simulink model "VVI"  (R2022a)
settings: Solver=FixedStepAuto  StartTime=0.0  StopTime=50  FixedStep=1e-3  RelTol=1e-3  EnableMultiTasking=on
undefined symbols (not defined in the file): D1, D10, D11, D12, D13, D2, D3, D5, D8, D9, PTA0, PTA1, PTA2, PTB9, PTC17, PTC4, PTD0, PTD1, PTD2, PTD3
libraries: frdmk64flib x10
settings Model: ExtModeTrigDuration=5  Creator=tygre  LastModifiedBy=MichaelGolendukhin
settings OptimizationCC: EnhancedBackFolding=on  PassReuseOutputArgsAs=Individual arguments  ZeroExternalMemoryAtStartup=off  ZeroInternalMemoryAtStartup=off  MaxStackSize=64  OptimizeBlockOrder=speed  DifferentSizesBufferReuse=on  OptimizationCustomize=off  EfficientTunableParamExpr=on
settings DebuggingCC: ParameterTunabilityLossMsg=error
settings HardwareCC: ProdBitPerPointer=32  ProdBitPerSizeT=32  ProdBitPerPtrDiffT=32  ProdLargestAtomicInteger=Long  ProdLargestAtomicFloat=Double  ProdWordSize=32  ProdHWDeviceType=ARM Compatible->ARM Cortex  UseEmbeddedCoderFeatures=off
settings SFSimCC: MATLABDynamicMemAlloc=off
settings RTWCC: SystemTargetFile=ert.tlc  HardwareBoard=NXP FRDM-K64F  TLCOptions="-aInlineSetEventsForThisBaseRateFcn=TLC_FALSE -aSuppressMultiTaskScheduler=TLC_FALSE  -aRateBasedStepFcn=0"  TemplateMakefile=ert_default_tmf  Toolchain=GNU Tools for ARM Embedded Processors
settings CodeAppCC: ForceParamTrailComments=on  IgnoreCustomStorageClasses=off  OperatorAnnotations=on  SimulinkDataObjDesc=on  SFDataObjDesc=on  InsertBlockDesc=on
settings ERTTargetCC: SupportNonInlinedSFcns=on  ExtModeTransport=4  ExtModeMexFile=sendToCommService

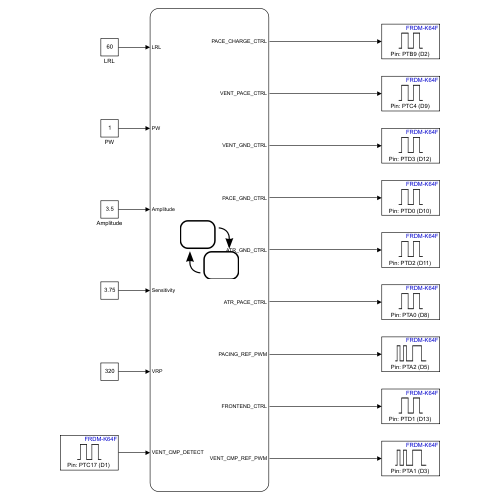
[thumbnail: Simulink's stored preview of the top-level diagram]
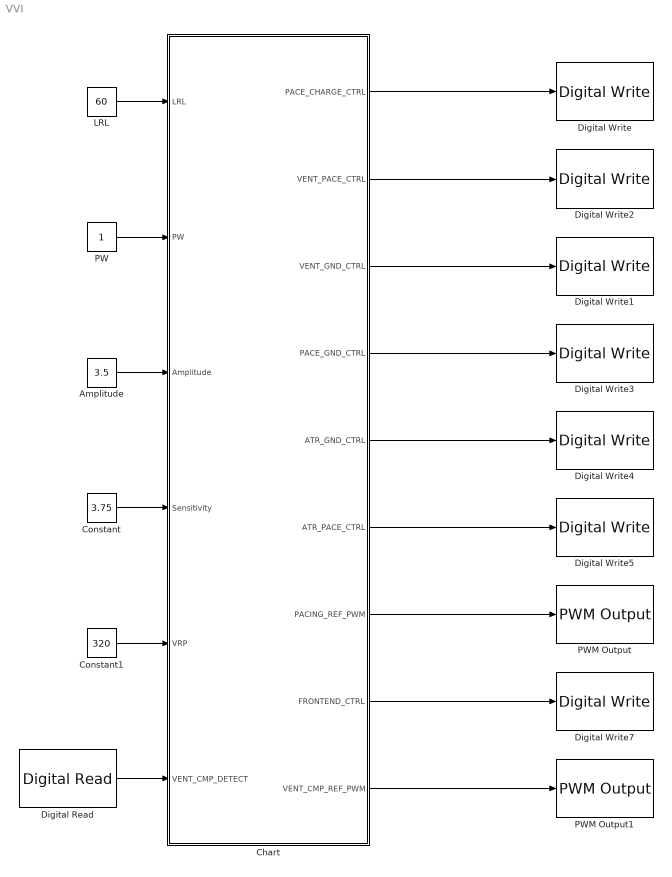
== system VVI ==
  Amplitude : Constant  Value=3.5  OutDataTypeStr=double
  Chart : Stateflow chart  TreatAsAtomicUnit=on
  Constant : Constant  Value=3.75
  Constant1 : Constant  Value=320
  Digital Read : frdmk64flib/Digital Read  Whichpin=PTC17 (D1)  SampleTime=-1
  Digital Write : frdmk64flib/Digital Write  Whichpin=PTB9 (D2)
  Digital Write1 : frdmk64flib/Digital Write  Whichpin=PTD3 (D12)
  Digital Write2 : frdmk64flib/Digital Write  Whichpin=PTC4 (D9)
  Digital Write3 : frdmk64flib/Digital Write  Whichpin=PTD0 (D10)
  Digital Write4 : frdmk64flib/Digital Write  Whichpin=PTD2 (D11)
  Digital Write5 : frdmk64flib/Digital Write  Whichpin=PTA0 (D8)
  Digital Write7 : frdmk64flib/Digital Write  Whichpin=PTD1 (D13)
  LRL : Constant  Value=60
  PW : Constant
  PWM Output : frdmk64flib/PWM Output  Whichpin=PTA2 (D5)  InitialFrequency=2000  InitialDutyCycle=0
  PWM Output1 : frdmk64flib/PWM Output  Whichpin=PTA1 (D3)  InitialFrequency=2000  InitialDutyCycle=0
  wires:
  LRL/1 -> Chart/1(LRL)
  PW/1 -> Chart/2(PW)
  Amplitude/1 -> Chart/3(Amplitude)
  Chart/1(PACE_CHARGE_CTRL) -> Digital Write/1
  Chart/2(VENT_PACE_CTRL) -> Digital Write2/1
  Chart/3(VENT_GND_CTRL) -> Digital Write1/1
  Chart/4(PACE_GND_CTRL) -> Digital Write3/1
  Chart/5(ATR_GND_CTRL) -> Digital Write4/1
  Chart/6(ATR_PACE_CTRL) -> Digital Write5/1
  Chart/7(PACING_REF_PWM) -> PWM Output/1
  Constant/1 -> Chart/4(Sensitivity)
  Constant1/1 -> Chart/5(VRP)
  Chart/8(FRONTEND_CTRL) -> Digital Write7/1
  Chart/9(VENT_CMP_REF_PWM) -> PWM Output1/1
  Digital Read/1 -> Chart/6(VENT_CMP_DETECT)

== stateflow chart VVI/Chart ==
  state VVI_Charging_C22
    entry:
    ATR_PACE_CTRL = false;
    VENT_PACE_CTRL = false;
    PACING_REF_PWM = Amplitude * 20;
    PACE_CHARGE_CTRL = true;
    PACE_GND_CTRL = true;
    ATR_GND_CTRL = false;
    VENT_GND_CTRL = true;
  state VVI_Pacing
    entry:
    PACE_CHARGE_CTRL = false;
    PACE_GND_CTRL = true;
    ATR_PACE_CTRL = false;
    ATR_GND_CTRL = false;
    VENT_GND_CTRL = false;
    VENT_PACE_CTRL = true;
  state VVI_Sensing
    entry:
    FRONTEND_CTRL = true;
    VENT_CMP_REF_PWM = (Sensitivity)*20;
    exit:
    FRONTEND_CTRL = false;
  (default) -> VVI_Charging_C22
  VVI_Pacing -> VVI_Charging_C22 : after (PW, msec)
  VVI_Sensing -> VVI_Charging_C22 [order 2] : [VENT_CMP_DETECT == true]
  VVI_Charging_C22 -> VVI_Sensing : after(VRP, msec)
  VVI_Sensing -> VVI_Pacing [order 1] : after(((60000/LRL) - VRP), msec)
  data: PACE_CHARGE_CTRL output boolean; VENT_PACE_CTRL output boolean; VENT_GND_CTRL output boolean; PACE_GND_CTRL output boolean; LRL input double; PW input double; Amplitude input double; ATR_GND_CTRL output boolean; ATR_PACE_CTRL output boolean; PACING_REF_PWM output double; Sensitivity input double; VRP input double; FRONTEND_CTRL output boolean; VENT_CMP_REF_PWM output double; VENT_CMP_DETECT input boolean
